simulink model "sistema"  (R2023a)
settings: Solver=ode23t  StartTime=0.0  StopTime=100  RelTol=1e-3
settings Model: Creator=Bricia Arellano  LastModifiedBy=Bricia Arellano
settings DataIOCC: ReturnWorkspaceOutputs=off  TimeSaveName=t
settings DebuggingCC: AlgebraicLoopMsg=none  ArtificialAlgebraicLoopMsg=none  MaxConsecutiveZCsMsg=none  ModelReferenceExtraNoncontSigs=none  OperatingPointInterfaceChecksumMismatchMsg=none

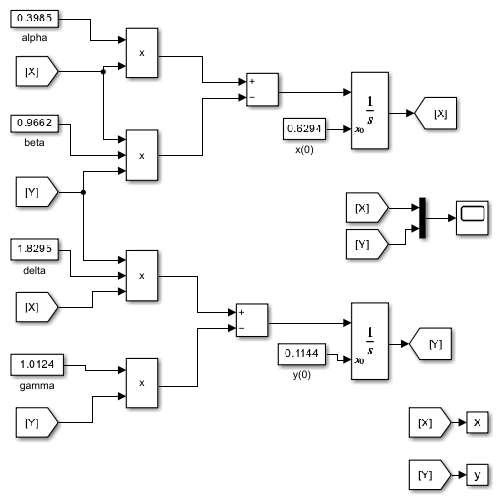
[thumbnail: Simulink's stored preview of the top-level diagram]
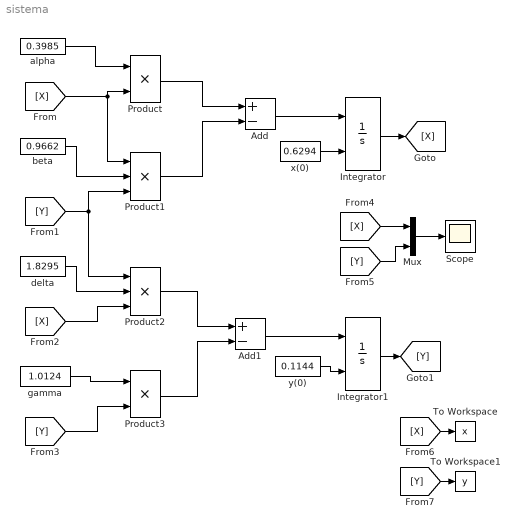
== system sistema ==
  Add : Sum  Inputs=+-
  Add1 : Sum  Inputs=+-
  Integrator : Integrator  InitialConditionSource=external
  Integrator1 : Integrator  InitialConditionSource=external
  Mux : Mux  Inputs=2
  Product : Product
  Product1 : Product  Inputs=3
  Product2 : Product  Inputs=3
  Product3 : Product
  Scope : Scope
  To Workspace : ToWorkspace  VariableName=x  SampleTime=-1
  To Workspace1 : ToWorkspace  VariableName=y  SampleTime=-1
  alpha : Constant  Value=0.3985
  beta : Constant  Value=0.9662
  delta : Constant  Value=1.8295
  gamma : Constant  Value=1.0124
  x(0) : Constant  Value=0.6294
  y(0) : Constant  Value=0.1144
  wires:
  alpha/1 -> Product/1
  [X] -> Product1/1, Product/2
  Mux/1 -> Scope/1
  beta/1 -> Product1/2
  [Y] -> Product2/1, Product1/3
  [X] -> Mux/1
  [Y] -> Mux/2
  delta/1 -> Product2/2
  [X] -> Product2/3
  gamma/1 -> Product3/1
  [Y] -> Product3/2
  x(0)/1 -> Integrator/2
  y(0)/1 -> Integrator1/2
  Integrator/1 -> [X]
  Integrator1/1 -> [Y]
  [X] -> To Workspace/1
  [Y] -> To Workspace1/1
  Product/1 -> Add/1
  Product1/1 -> Add/2
  Product2/1 -> Add1/1
  Product3/1 -> Add1/2
  Add1/1 -> Integrator1/1
  Add/1 -> Integrator/1
